simulink model "soccerVision"  (R2017b)
settings: Solver=VariableStepAuto  StartTime=0.0  StopTime=10.0  RelTol=1e-3
InitFcn:
  | visionConfiguration;
model workspace (MATLAB code in the model file):
  | visionConfiguration;
values from neighbouring files (symbols this model uses):
  clusterProximityThreshold = 0.05    [loadRobot.m]    (also in soccer_vision_setup.m; visionConfiguration.m)
  netAngleThreshold = pi/10    (= 0.314159265359)    [loadRobot.m]    (also in soccer_vision_setup.m; visionConfiguration.m)
  scalerho = 1/500    (= 0.002)    [loadRobot.m]    (also in soccer_vision_setup.m; visionConfiguration.m)
undefined symbols (not defined in the file or in its folder): gray
libraries: visiontransforms x2, visiontextngfix x1, visionanalysis x1, visionstatistics x1, dspvision x1
settings Model: Creator=vuwij  LastModifiedBy=vuwij

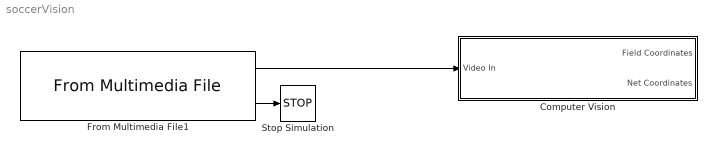
== system soccerVision ==
  Computer Vision : Subsystem
  From Multimedia File1 : dspvision/From Multimedia File  inputFilename=/Users/vuwij/Google Drive/Documents/2018 May/UTRA RoboSoccer/3. Software/soccer-matlab/soccer-vision/media/videos/2.mp4  loop=on  numPlays=1  outputStreams=Video only  videoDataType=single  audioDataType=int16  inheritSampleTime=on  userDefinedSampleTime=0.1  noAudioOutput=off  isIntensityVideo=off  fourcc=Intensity  colorVideoFormat=One multidimensional signal  outputEOF=on  dataOrg=Column-major  audioFrameSize=1024  computeAudioFrameSize=off  outSamplingMode=Sample based
      settings: SourceProductBaseCode=VP
  Stop Simulation : Stop
  wires:
  From Multimedia File1/2 -> Stop Simulation/1
  From Multimedia File1/1 -> Computer Vision/1(Video In)

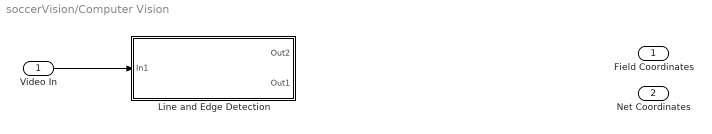
== system soccerVision/Computer Vision ==
  Video In : Inport
  Line and Edge Detection : Subsystem
  Field Coordinates : Outport
  Net Coordinates : Outport  Port=2
  wires:
  Video In/1 -> Line and Edge Detection/1(In1)

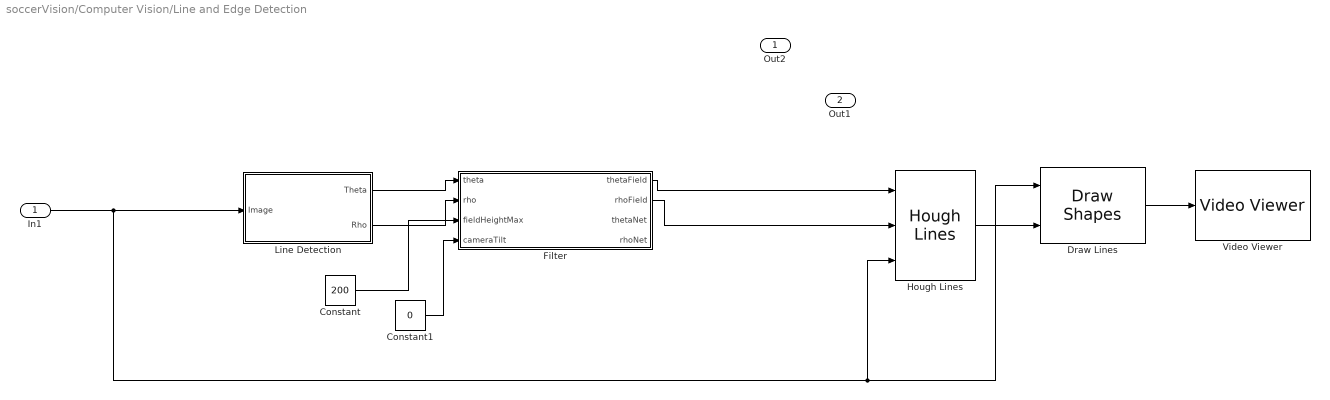
== system soccerVision/Computer Vision/Line and Edge Detection ==
  In1 : Inport
  Constant : Constant  Value=200
  Constant1 : Constant  Value=0
  Draw Lines : visiontextngfix/Draw Shapes  shape=Lines  fill=off  lineWidth=15  fillClrSource=Specify via dialog  display=Black  intensity=200  color=[0 128 0]  opacity=0.6  viewport=Entire image  antialiasing=off  inType=Obsolete  imagePorts=One multidimensional signal  prodOutputMode=Binary point scaling  prodOutputWordLength=32  prodOutputFracLength=14  memoryMode=Specify word length  memoryWordLength=16  memoryFracLength=14  roundingMode=Floor  overflowMode=off
      settings: SourceProductName=Computer Vision System Toolbox
  Filter : MATLAB Function  TreatAsAtomicUnit=on
  Hough Lines : visiontransforms/Hough Lines  sineCompMethod=Trigonometric function  thetaRes=pi/180  firstCoeffMode=Specify word length  firstCoeffWordLength=16  firstCoeffFracLength=15  prodOutputMode=Binary point scaling  prodOutputWordLength=32  prodOutputFracLength=16  roundingMode=Nearest  overflowMode=on
      settings: SourceProductName=Computer Vision System Toolbox  SourceProductBaseCode=VP
  Line Detection : Subsystem
  Video Viewer : VideoViewer  colormapValue=gray(256)  FigPos=[876 769 905 574]
  Out2 : Outport
  Out1 : Outport  Port=2
  wires:
  Filter/1(thetaField) -> Hough Lines/1
  Draw Lines/1 -> Video Viewer/1
  In1/1 -> Draw Lines/1, Hough Lines/3, Line Detection/1(Image)
  Filter/2(rhoField) -> Hough Lines/2
  Hough Lines/1 -> Draw Lines/2
  Line Detection/1(Theta) -> Filter/1(theta)
  Line Detection/2(Rho) -> Filter/2(rho)
  Constant/1 -> Filter/3(fieldHeightMax)
  Constant1/1 -> Filter/4(cameraTilt)

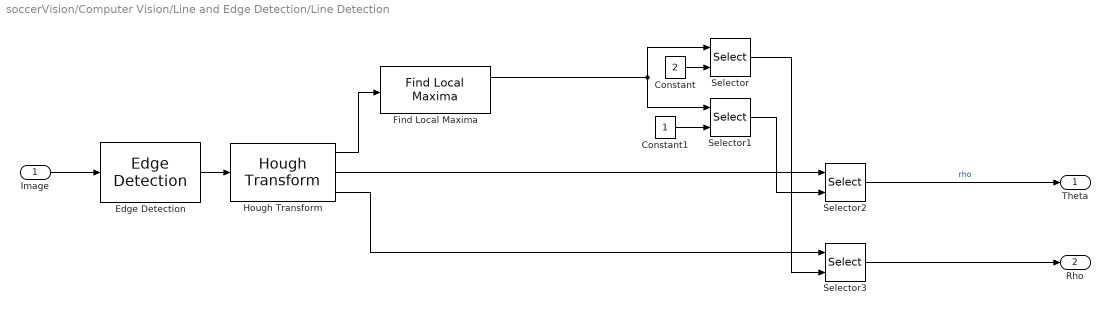
== system soccerVision/Computer Vision/Line and Edge Detection/Line Detection ==
  Image : Inport
  Constant : Constant  Value=2
  Constant1 : Constant
  Edge Detection : visionanalysis/Edge Detection  method=Sobel  outputType=Binary image  userDefinedThreshold=off  thresholdSource=Input port  threshold=20  thresholdTuning=5  edgeThinning=off  threshold_canny=[0.25 0.60]  autoPercent=70  sigma=1  prodOutputMode=Binary point scaling  prodOutputWordLength=32  prodOutputFracLength=8  roundingMode=Floor  overflowMode=off
      settings: SourceProductName=Computer Vision System Toolbox  SourceProductBaseCode=VP
  Find Local Maxima : visionstatistics/Find Local Maxima  num_peaks=20  nhood_size=[5 7]  src_thresh=Obsolete9b  src_thresh_inuse=Specify via dialog  threshold=10  inputIsHough=on  dt_peak=uint32  isOutVarDim=off  dt_count=uint32
      settings: SourceProductName=Computer Vision System Toolbox  SourceProductBaseCode=VP
  Hough Transform : visiontransforms/Hough Transform  theta_res=pi/360  rho_res=1  out_theta_rho=on  outdtmode=double  firstCoeffMode=Binary point scaling  firstCoeffWordLength=16  firstCoeffFracLength=14  secondCoeffMode=Binary point scaling  secondCoeffWordLength=32  secondCoeffFracLength=16  outputMode=Binary point scaling  outputWordLength=16  outputFracLength=0  accumMode=Binary point scaling  accumWordLength=32  accumFracLength=20  prodOutputMode=Binary point scaling  prodOutputWordLength=32  prodOutputFracLength=20  memoryMode=Binary point scaling  memoryWordLength=32  memoryFracLength=16  roundingMode=Nearest  overflowMode=on
      settings: SourceProductName=Computer Vision System Toolbox  SourceProductBaseCode=VP
  Selector : Selector  NumberOfDimensions=2  InputPortWidth=2  IndexOptions=Select all,Index vector (port)  Indices=1,1  OutputSizes=1,1
  Selector1 : Selector  NumberOfDimensions=2  InputPortWidth=2  IndexOptions=Select all,Index vector (port)  Indices=0,1  OutputSizes=1,1
  Selector2 : Selector  NumberOfDimensions=2  InputPortWidth=3  IndexOptions=Select all,Index vector (port)  Indices=[1 3],1  OutputSizes=1,1
  Selector3 : Selector  NumberOfDimensions=2  InputPortWidth=3  IndexOptions=Select all,Index vector (port)  Indices=[1 3],1  OutputSizes=1,1
  Theta : Outport
  Rho : Outport  Port=2
  wires:
  Constant/1 -> Selector/2
  Hough Transform/1 -> Find Local Maxima/1
  Hough Transform/2 -> Selector2/1
  Constant1/1 -> Selector1/2
  Find Local Maxima/1 -> Selector1/1, Selector/1
  Selector/1 -> Selector3/2
  Selector1/1 -> Selector2/2
  Edge Detection/1 -> Hough Transform/1
  Hough Transform/3 -> Selector3/1
  Selector2/1 -> Theta/1  "rho"
  Image/1 -> Edge Detection/1
  Selector3/1 -> Rho/1

== matlab function soccerVision/Computer Vision/Line and Edge Detection/Filter ==
  data: thetaField output; theta input; rhoField output; rho input; thetaNet output; rhoNet output; fieldHeightMax input; cameraTilt input; scalerho parameter; clusterProximityThreshold parameter; netAngleThreshold parameter
function [thetaField, rhoField, thetaNet, rhoNet]  = filterLines(theta, rho, fieldHeightMax, cameraTilt, scalerho, clusterProximityThreshold, netAngleThreshold)
    % Fix the negative lines
    lines = [transpose(theta),transpose(rho) * scalerho];
    for i = 1:length(lines)
       if lines(i,2) < 0
          lines(i,1) = lines(i,1) + pi;
          lines(i,2) = -lines(i,2);
       end
       if lines(i,1) > pi
          lines(i,1) = lines(i,1) - 2 * pi; 
       end
    end
    
    sumdbest = 1000000;
    kbest = 0;
    linesFilteredBest = 0;
    
    % Proper clustering
    for k=1:6
        [~,C,sumd] = kmeans(lines,k,'Replicates',1);
        tooclose = 0;
        for i = 1:k
            for j = 1:k
                if i == j 
                    continue;
                end
                if(norm(C(i,:)-C(j,:)) < clusterProximityThreshold)
                    tooclose = 1;
                end
            end
        end
        
        if(tooclose == 1)
            continue
        end
        
        if (mean(sumd) < sumdbest)
            sumdbest = mean(sumd);
            kbest = k;
            linesFilteredBest = C;
        end
    end
   

    
    % Plot the data
%     plot(lines(:,1),lines(:,2), 'o')
%     hold on;
%     plot(linesFilteredBest(:,1),linesFilteredBest(:,2), 'x')
%     title 'Rho and theta data data for lines'
%     xlabel 'Theta'
%     ylabel 'Rho'
%     xlim([-pi pi])
%     ylim([0 640 * scalerho])
%     grid minor
%     hold off;
    
    % Figure out which is part of the field
    thetaField = zeros(1,6);
    rhoField = zeros(1,6);
    thetaNet = zeros(1,6);
    rhoNet = zeros(1,6);
    fieldLineCount = 0;
    netLineCount = 0;
    
    for i = 1:kbest
        if (linesFilteredBest(i,1) < netAngleThreshold + cameraTilt && linesFilteredBest(i,1) > -netAngleThreshold + cameraTilt)
            netLineCount = netLineCount + 1;
            thetaNet(netLineCount) = transpose(linesFilteredBest(i,1));
            rhoNet(netLineCount) = transpose(linesFilteredBest(i,2)) / scalerho;
        else
            %Todo fix this so thresholding properly
           if linesFilteredBest(i,2) > fieldHeightMax * scalerho || (linesFilteredBest(i,1) < 0 && linesFilteredBest(i,1) > - pi/3)
               fieldLineCount = fieldLineCount + 1;
               thetaField(fieldLineCount) = transpose(linesFilteredBest(i,1));
               rhoField(fieldLineCount) = transpose(linesFilteredBest(i,2)) / scalerho;
           end
        end
    end  
end
